simulink model "inner_PID_position_d"  (R2016a)
settings: Solver=VariableStepAuto  StartTime=0.0  StopTime=50  RelTol=1e-3
settings Model: Creator=Daniel  LastModifiedBy=mgreiff
settings DataIOCC: LimitDataPoints=on
settings DebuggingCC: AllowSymbolicDim=off
settings ModelReferenceCC: PropagateSignalLabelsOutOfModel=off
settings GRTTargetCC: GeneratePreprocessorConditionals=Use local settings

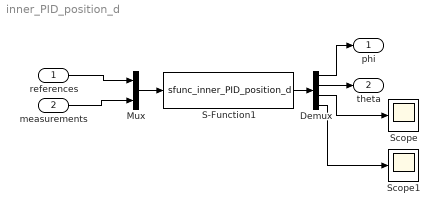
== system inner_PID_position_d ==
  references : Inport  PortDimensions=12
  measurements : Inport  Port=2  PortDimensions=12
  Demux : Demux
  Mux : Mux  Inputs=2
  S-Function1 : S-Function  FunctionName=sfunc_inner_PID_position_d  Parameters=PD_position_param  SFunctionDeploymentMode=off  EnableBusSupport=off
  Scope : Scope
  Scope1 : Scope
  phi : Outport
  theta : Outport  Port=2
  wires:
  measurements/1 -> Mux/2
  references/1 -> Mux/1
  Mux/1 -> S-Function1/1
  S-Function1/1 -> Demux/1
  Demux/1 -> phi/1
  Demux/2 -> theta/1
  Demux/3 -> Scope/1
  Demux/4 -> Scope1/1
